simulink model "Ex2_2"  (Simulink 6.0)
settings: Solver=FixedStepDiscrete  StartTime=0.0  StopTime=Tstop*10  FixedStep=1  RelTol=1e-3
values from neighbouring files (symbols this model uses):
  c10 = -0.1    [Ex2_2launch.m]
  c2 = -0.01    [Ex2_2launch.m]
  c3 = 0.01    [Ex2_2launch.m]
  c4 = 0.001    [Ex2_2launch.m]
  c5 = 0.1    [Ex2_2launch.m]
  c6 = -0.01    [Ex2_2launch.m]
  c7 = 0.01    [Ex2_2launch.m]
  c8 = 0.1    [Ex2_2launch.m]
  c9 = 0.001    [Ex2_2launch.m]
  infreq = 2311/Npoint    (= 0.141043637473)    [Ex2_2launch.m]
  N = 14    [Ex2_2launch.m]    (also in Ex2_3launch.m = 12)
  Npoint = 2^14+1    (= 16385)    [Ex2_2launch.m]    (also in Ex2_3launch.m = 16384)
libraries: simulink x1, dspsnks4 x1, dng_gmslib x1
settings Model: Creator=francomaloberti  LastModifiedBy=Cri  ExtModeAutoUpdateStatusClock=off
settings DataIOCC: SignalLoggingName=sigsOut
settings DebuggingCC: SolverPrmCheckMsg=none
settings HardwareCC: TargetUnknown=on

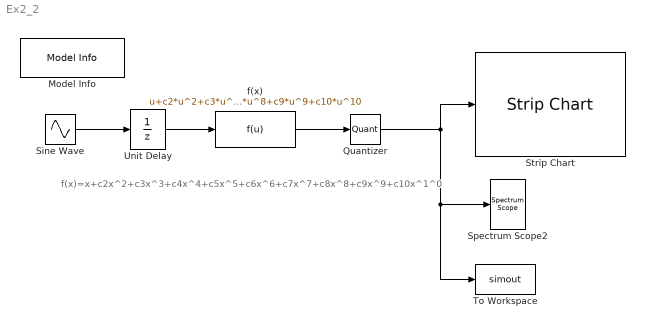
== system Ex2_2 ==
  note: f(x)=x+c2x^2+c3x^3+c4x^4+c5x^5+c6x^6+c7x^7+c8x^8+c9x^9+c10x^1^0
  Model Info : simulink/Model-Wide Utilities/Model Info  InitialBlockCM=None  BlockCM=None  Frame=on  DisplayStringWithTags=Example 2.2 page 65  HorizontalTextAlignment=Center  LeftAlignmentValue=0.5  SourceBlockDiagram=Ex2_2  TagMaxNumber=20
  Quantizer : Quantizer  QuantizationInterval=1/2^N
  Sine Wave : Sin  Frequency=2*pi*infreq  SampleTime=0
  Spectrum Scope2 : dspsnks4/Spectrum Scope  ScopeProperties=off  Domain=Frequency  HorizSpan=1  UseBuffer=on  BufferSize=(Npoint-1)/4  Overlap=2  inpFftLenInherit=on  FFTlength=Npoint-1  numAvg=2  DisplayProperties=on  AxisGrid=on  Memory=on  FrameNumber=on  AxisLegend=off  AxisZoom=off  OpenScopeAtSimStart=on  OpenScopeImmediately=off  FigPos=[100 100 600 400]  AxisProperties=off  XUnits=Hertz  XRange=[0...Fs/2]  InheritXIncr=off  XIncr=1.0  XLabel=Samples  YUnits=dB  YLabel=Magnitude, dB  LineProperties=off  LineDisables=on  LineStyles=-  LineColors=[0 0 1]
      link override Periodogram: winsamp=Periodic  inheritFFT=off  wintype=Blackman
      settings: YMin=-160  YMax=20
  Strip Chart : dng_gmslib/Strip Chart/Strip Chart  Tag=000  progid=mwStrip.stripctrl.1  connect=input  init="hActx.XTicMode = 1;hActx.XSpan = 10/60/60/24; hActx.TimeSecondsFormat = '%M:%S'; hActx.TimeDateFormat = ''; hActx.TimeDaysFormat = ''; hActx.TimeHoursFormat = ''; hActx.TimeMinutesFormat = ''; hActx.TimeMonthsFormat = ''; hActx.TimeYearsFormat = ''; % Set x-axis to display time; set span = 10 sec (in fixed units=days); set display format = \"min:sec\" only"  inblock=on  border=on  dialOut=0  updateParam=0
  To Workspace : ToWorkspace  VariableName=simout  SampleTime=-1  SaveFormat=Array
  Unit Delay : UnitDelay
  f(x) : Fcn  Expr=u+c2*u^2+c3*u^3+c4*u^4+c5*u^5+c6*u^6+c7*u^7+c8*u^8+c9*u^9+c10*u^10
  wires:
  Unit Delay/1 -> f(x)/1
  f(x)/1 -> Quantizer/1
  Quantizer/1 -> To Workspace/1, Spectrum Scope2/1, Strip Chart/1
  Sine Wave/1 -> Unit Delay/1
